simulink model "fsr_ut"  (Simulink 8.1)
settings: Solver=FixedStepDiscrete  StartTime=0.0  StopTime=Inf  FixedStep=0.005  RelTol=1e-3
libraries: siltestlib x2, fsr x1
settings Model: Creator=xsellart  LastModifiedBy=AT015555
settings DataIOCC: SignalLoggingSaveFormat=Dataset
settings OptimizationCC: ExpressionDepthLimit=128
settings DebuggingCC: FcnCallInpInsideContextMsg=EnableAllAsError
settings GRTTargetCC: CombineOutputUpdateFcns=on  GRTInterface=off

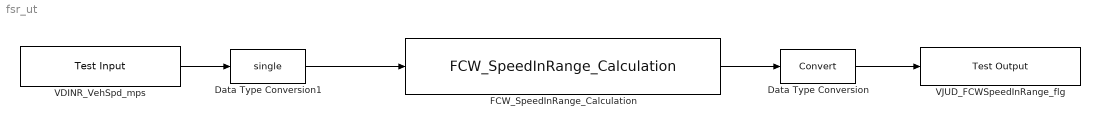
== system fsr_ut ==
  Data Type Conversion : DataTypeConversion
  Data Type Conversion1 : DataTypeConversion  OutDataTypeStr=single
  FCW_SpeedInRange_Calculation : fsr/FCW_SpeedInRange_Calculation
  VDINR_VehSpd_mps : siltestlib/Test Input  varname=VDINR_VehSpd_mps  sampletime=0.005
  VJUD_FCWSpeedInRange_flg : siltestlib/Test Output  varname=VJUD_FCWSpeedInRange_flg  sampletime=-1
  wires:
  VDINR_VehSpd_mps/1 -> Data Type Conversion1/1
  FCW_SpeedInRange_Calculation/1 -> Data Type Conversion/1
  Data Type Conversion/1 -> VJUD_FCWSpeedInRange_flg/1
  Data Type Conversion1/1 -> FCW_SpeedInRange_Calculation/1
